simulink subsystem "PowerSplitDriveUnitBasic_refsub"  (R2021a)
settings: Solver=VariableStepAuto  StartTime=0.0  StopTime=10.0  RelTol=1e-3
libraries: nesl_utility x3
settings Model: Creator=isaacito  LastModifiedBy=isaacito
settings SolverCC: AlgebraicLoopSolver=TrustRegion
settings DebuggingCC: SFMachineParentedDataDiag=warning

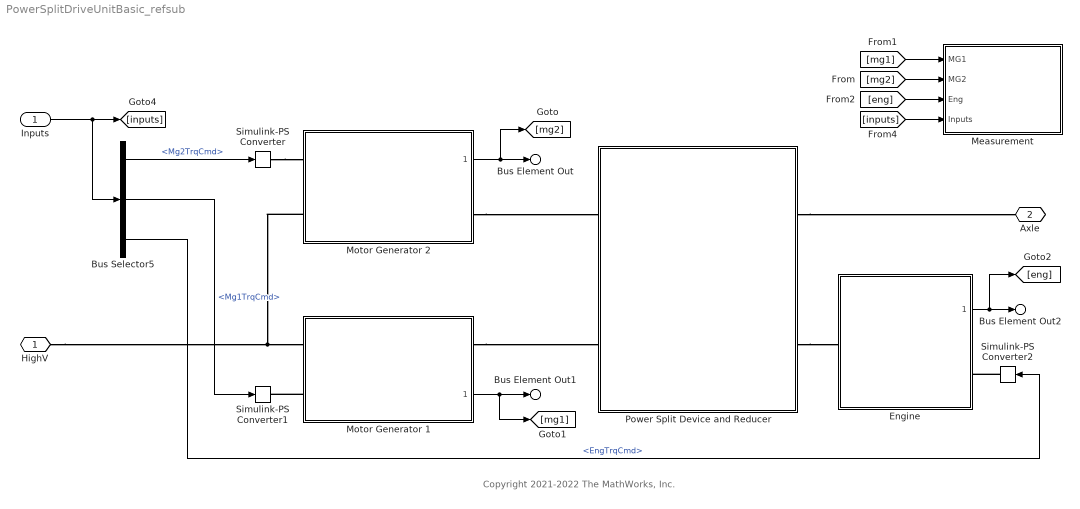
== system PowerSplitDriveUnitBasic_refsub ==
  note: Copyright 2021-2022 The MathWorks, Inc.
  Inputs : Inport
  Bus Selector5 : BusSelector  OutputSignals=Mg2TrqCmd,Mg1TrqCmd,EngTrqCmd
  Engine : Subsystem  ReferencedSubsystem=EngineCustom_refsub
  Measurement : Subsystem
  Motor Generator 1 : Subsystem  ReferencedSubsystem=MotorGenerator1Basic_refsub
      settings: PortSchema="{\"entries\":[{\"content\":{\"sides\":[{\"content\":{\"connectorIds\":[\"LConn1\",\"LConn2\"]},\"type\":\"ConnectorPlacement.EquallySpacedRectSide\",\"uuid\":\"3f13e6b9-9785-470e-b4e7-2230544192d3\"},{\"content\":{\"connectorIds\":[\"RConn1\",\"Out1\"],\"side\":\"RIGHT\"},\"type\":\"ConnectorPlacement.EquallySpacedRectSide\",\"uuid\":\"c86dc6d1-f3ea-46c4-b113-258136dcfee4\"},{\"content\":{\"connectorIds\":[],\"side\":\"TOP\"},\"type\":\"ConnectorPlacement.EquallySpacedRectSide\",\"uuid\":\"633c827b-a9f1-4506-b379-ba2a2b41c3a4\"},{\"content\":{\"connectorIds\":[],\"side\":\"HIDDEN\"},\"type\":\"ConnectorPlacement.EquallySpacedRectSide\",\"uuid\":\"493696b9-c4b5-4599-b165-b63d9ea3db6c\"}]},\"type\":\"ConnectorPlacement.EquallySpacedConnector\",\"uuid\":\"29b0ca39-3f61-4a79-b1ec-51b22406ccf5\"}],\"packageUris\":[\"http://schema.mathworks.com/mf0/Connector/R2020b\"],\"version\":\"1.0\"}"
  Motor Generator 2 : Subsystem  ReferencedSubsystem=MotorGenerator2Basic_refsub
      settings: PortSchema="{\"entries\":[{\"content\":{\"sides\":[{\"content\":{\"connectorIds\":[\"LConn2\",\"LConn1\"]},\"type\":\"ConnectorPlacement.EquallySpacedRectSide\",\"uuid\":\"fb1ae627-2a11-4cdc-b40f-1f1ad643affe\"},{\"content\":{\"connectorIds\":[\"Out1\",\"RConn1\"],\"side\":\"RIGHT\"},\"type\":\"ConnectorPlacement.EquallySpacedRectSide\",\"uuid\":\"00f90b97-65a5-4f07-9d46-c4d934bbcebd\"},{\"content\":{\"connectorIds\":[],\"side\":\"TOP\"},\"type\":\"ConnectorPlacement.EquallySpacedRectSide\",\"uuid\":\"1403ad56-fcb4-428e-96ec-7b36e4f507b4\"},{\"content\":{\"connectorIds\":[],\"side\":\"HIDDEN\"},\"type\":\"ConnectorPlacement.EquallySpacedRectSide\",\"uuid\":\"421b449c-9b3e-4f4b-a79f-ec7613821770\"}]},\"type\":\"ConnectorPlacement.EquallySpacedConnector\",\"uuid\":\"1887aacf-d3d5-4d1b-946b-79f82bd43283\"}],\"packageUris\":[\"http://schema.mathworks.com/mf0/Connector/R2020b\"],\"version\":\"1.0\"}"
  Power Split Device and Reducer : Subsystem  ReferencedSubsystem=PowerSplitGeartrainBasic_refsub
  Simulink-PS Converter : nesl_utility/Simulink-PS Converter  PhysicalDomain=network_engine_domain  SubClassName=ps_input  LeftPortType=input  RightPortType=output  PseudoPeriodic=off  Frequencies=[]  NoiseDistribution=none  NoiseParameters=[]  Unit=N*m  AffineConversion=off  FilteringAndDerivatives=provide  SimscapeFilterOrder=1  InputFilterTimeConstant=0.001  UdotUserProvided=0
  Simulink-PS Converter1 : nesl_utility/Simulink-PS Converter  PhysicalDomain=network_engine_domain  SubClassName=ps_input  LeftPortType=input  RightPortType=output  PseudoPeriodic=off  Frequencies=[]  NoiseDistribution=none  NoiseParameters=[]  Unit=N*m  AffineConversion=off  FilteringAndDerivatives=provide  SimscapeFilterOrder=1  InputFilterTimeConstant=0.001  UdotUserProvided=0
  Simulink-PS Converter2 : nesl_utility/Simulink-PS Converter  PhysicalDomain=network_engine_domain  SubClassName=ps_input  LeftPortType=input  RightPortType=output  PseudoPeriodic=off  Frequencies=[]  NoiseDistribution=none  NoiseParameters=[]  Unit=N*m  AffineConversion=off  FilteringAndDerivatives=provide  SimscapeFilterOrder=1  InputFilterTimeConstant=0.001  UdotUserProvided=0
  HighV : PMIOPort  Side=Left
  Axle : PMIOPort  Port=2  Side=Right
  Bus Element Out : Outport  PortName=Info  Element=mg2
  Bus Element Out1 : Outport  PortName=Info  Element=mg1
  Bus Element Out2 : Outport  PortName=Info  Element=eng
  wires:
  Motor Generator 2/1 -> Bus Element Out/1, [mg2]
  Motor Generator 1/1 -> Bus Element Out1/1, [mg1]
  Engine/1 -> Bus Element Out2/1, [eng]
  Bus Selector5/3 -> Simulink-PS Converter2/1  "<EngTrqCmd>"
  Bus Selector5/2 -> Simulink-PS Converter1/1  "<Mg1TrqCmd>"
  Inputs/1 -> [inputs], Bus Selector5/1
  Bus Selector5/1 -> Simulink-PS Converter/1  "<Mg2TrqCmd>"
  [mg2] -> Measurement/2(MG2)
  [mg1] -> Measurement/1(MG1)
  [eng] -> Measurement/3(Eng)
  [inputs] -> Measurement/4(Inputs)
  connections:
  Motor Generator 2/LConn1 -- HighV/RConn1 -- Motor Generator 1/LConn1
  Motor Generator 2/RConn1 -- Power Split Device and Reducer/LConn1
  Motor Generator 1/RConn1 -- Power Split Device and Reducer/LConn2
  Simulink-PS Converter/RConn1 -- Motor Generator 2/LConn2
  Motor Generator 1/LConn2 -- Simulink-PS Converter1/RConn1
  Power Split Device and Reducer/RConn1 -- Axle/RConn1
  Simulink-PS Converter2/RConn1 -- Engine/RConn1
  Power Split Device and Reducer/RConn2 -- Engine/LConn1

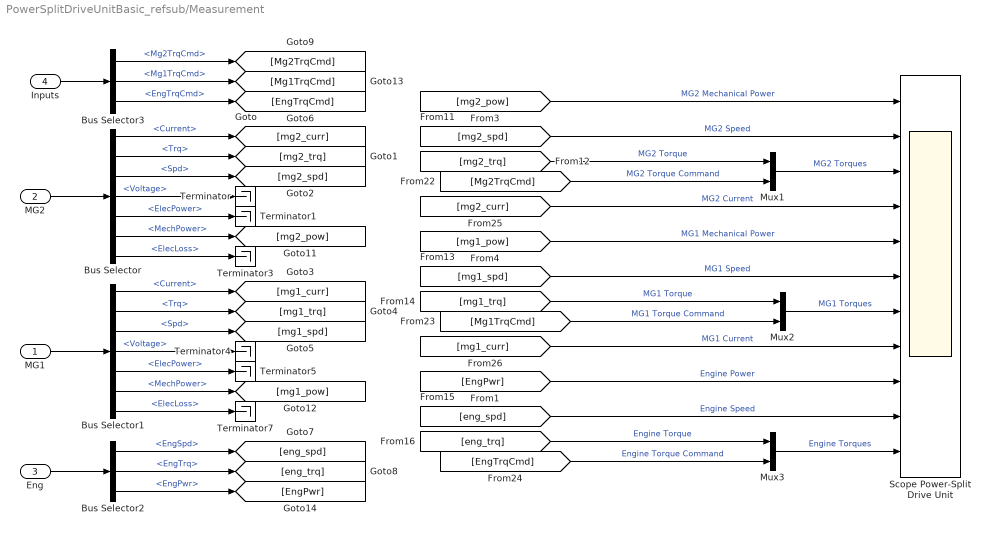
== system PowerSplitDriveUnitBasic_refsub/Measurement ==
  MG1 : Inport
  MG2 : Inport  Port=2
  Eng : Inport  Port=3
  Inputs : Inport  Port=4
  Bus Selector : BusSelector  OutputSignals=Current,Trq,Spd,Voltage,ElecPower,MechPower,ElecLoss
  Bus Selector1 : BusSelector  OutputSignals=Current,Trq,Spd,Voltage,ElecPower,MechPower,ElecLoss
  Bus Selector2 : BusSelector  OutputSignals=EngSpd,EngTrq,EngPwr
  Bus Selector3 : BusSelector  OutputSignals=Mg2TrqCmd,Mg1TrqCmd,EngTrqCmd
  Mux1 : Mux  Inputs=2
  Mux2 : Mux  Inputs=2
  Mux3 : Mux  Inputs=2
  Scope Power-Split Drive Unit : Scope  NumInputPorts=11
  Terminator{,1,3..5,7} (6 alike) : Terminator
  wires:
  [EngPwr] -> Scope Power-Split Drive Unit/9  "Engine Power"
  Bus Selector2/3 -> [EngPwr]  "<EngPwr>"
  [mg2_pow] -> Scope Power-Split Drive Unit/1  "MG2 Mechanical Power"
  [mg1_pow] -> Scope Power-Split Drive Unit/5  "MG1 Mechanical Power"
  Bus Selector1/4 -> Terminator4/1  "<Voltage>"
  Bus Selector1/7 -> Terminator7/1  "<ElecLoss>"
  Bus Selector1/6 -> [mg1_pow]  "<MechPower>"
  Bus Selector1/5 -> Terminator5/1  "<ElecPower>"
  Bus Selector/7 -> Terminator3/1  "<ElecLoss>"
  Bus Selector/6 -> [mg2_pow]  "<MechPower>"
  Bus Selector/5 -> Terminator1/1  "<ElecPower>"
  Bus Selector/4 -> Terminator/1  "<Voltage>"
  Mux3/1 -> Scope Power-Split Drive Unit/11  "Engine Torques"
  [eng_spd] -> Scope Power-Split Drive Unit/10  "Engine Speed"
  [mg1_curr] -> Scope Power-Split Drive Unit/8  "MG1 Current"
  Mux2/1 -> Scope Power-Split Drive Unit/7  "MG1 Torques"
  [mg1_spd] -> Scope Power-Split Drive Unit/6  "MG1 Speed"
  Bus Selector3/3 -> [EngTrqCmd]  "<EngTrqCmd>"
  Bus Selector3/2 -> [Mg1TrqCmd]  "<Mg1TrqCmd>"
  Bus Selector3/1 -> [Mg2TrqCmd]  "<Mg2TrqCmd>"
  Inputs/1 -> Bus Selector3/1
  Bus Selector2/2 -> [eng_trq]  "<EngTrq>"
  Bus Selector2/1 -> [eng_spd]  "<EngSpd>"
  Bus Selector1/3 -> [mg1_spd]  "<Spd>"
  Bus Selector1/2 -> [mg1_trq]  "<Trq>"
  Bus Selector1/1 -> [mg1_curr]  "<Current>"
  Bus Selector/3 -> [mg2_spd]  "<Spd>"
  Bus Selector/2 -> [mg2_trq]  "<Trq>"
  Bus Selector/1 -> [mg2_curr]  "<Current>"
  [mg2_spd] -> Scope Power-Split Drive Unit/2  "MG2 Speed"
  [eng_trq] -> Mux3/1  "Engine Torque"
  [mg2_curr] -> Scope Power-Split Drive Unit/4  "MG2 Current"
  [mg1_trq] -> Mux2/1  "MG1 Torque"
  [Mg1TrqCmd] -> Mux2/2  "MG1 Torque Command"
  [Mg2TrqCmd] -> Mux1/2  "MG2 Torque Command"
  Mux1/1 -> Scope Power-Split Drive Unit/3  "MG2 Torques"
  [mg2_trq] -> Mux1/1  "MG2 Torque"
  [EngTrqCmd] -> Mux3/2  "Engine Torque Command"
  Eng/1 -> Bus Selector2/1
  MG1/1 -> Bus Selector1/1
  MG2/1 -> Bus Selector/1
